simulink model "zad4popraw"  (R2023a)
settings: Solver=VariableStepAuto  StartTime=0.0  StopTime=10.0  RelTol=1e-3
values from neighbouring files (symbols this model uses):
  Gz = c2d(Gs,T,'zoh')    [zad1.m]
  L = [double(lx.l1); double(lx.l2); double(lx.l3)]    [zad6.m]
settings Model: Creator=pkutyl  LastModifiedBy=pkutyl

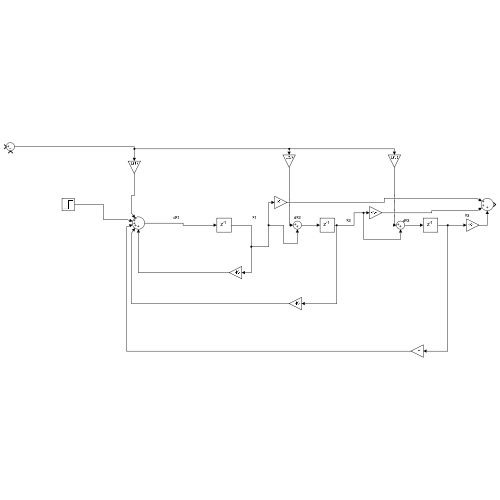
[thumbnail: Simulink's stored preview of the top-level diagram]
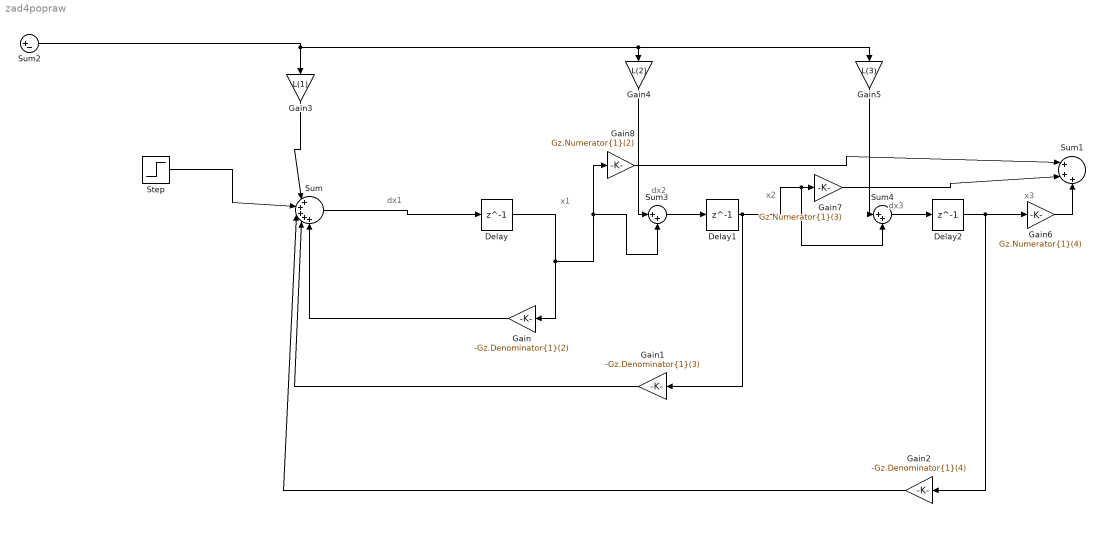
== system zad4popraw ==
  note: dx2
  note: x1
  note: dx3
  note: x3
  note: dx1
  note: x2
  Delay : Delay  DelayLength=1  InitialCondition=0
  Delay1 : Delay  DelayLength=1  InitialCondition=0
  Delay2 : Delay  DelayLength=1  InitialCondition=0
  Gain : Gain  Gain=-Gz.Denominator{1}(2)
  Gain1 : Gain  Gain=-Gz.Denominator{1}(3)
  Gain2 : Gain  Gain=-Gz.Denominator{1}(4)
  Gain3 : Gain  Gain=L(1)
  Gain4 : Gain  Gain=L(2)
  Gain5 : Gain  Gain=L(3)
  Gain6 : Gain  Gain=Gz.Numerator{1}(4)
  Gain7 : Gain  Gain=Gz.Numerator{1}(3)
  Gain8 : Gain  Gain=Gz.Numerator{1}(2)
  Step : Step  SampleTime=0
  Sum : Sum  Inputs=|+++++
  Sum1 : Sum  Inputs=|+++
  Sum2 : Sum  Inputs=|+-
  Sum3 : Sum  Inputs=|++
  Sum4 : Sum  Inputs=|++
  wires:
  Gain6/1 -> Sum1/3
  Gain7/1 -> Sum1/2
  Gain5/1 -> Sum4/1
  Step/1 -> Sum/2
  Gain2/1 -> Sum/3
  Sum2/1 -> Gain5/1, Gain4/1, Gain3/1
  Sum/1 -> Delay/1
  Delay1/1 -> Gain1/1, Sum4/2, Gain7/1
  Gain/1 -> Sum/5
  Sum3/1 -> Delay1/1
  Gain4/1 -> Sum3/1
  Gain1/1 -> Sum/4
  Sum4/1 -> Delay2/1
  Delay/1 -> Gain/1, Sum3/2, Gain8/1
  Delay2/1 -> Gain6/1, Gain2/1
  Gain3/1 -> Sum/1
  Gain8/1 -> Sum1/1
